simulink model "Tropfensimulation_x_y_Direction"  (R2025b)
settings: Solver=ode45  StartTime=0.0  StopTime=inf  RelTol=1e-6
values from neighbouring files (symbols this model uses):
  h0 = [0;3]    [Tropfensimulation_x_y_Direction_init.m]
  v0 = [7.5;0]    [Tropfensimulation_x_y_Direction_init.m]
libraries: simulink x1
settings Model: Creator=elmue  LastModifiedBy=ssokolov
settings SolverCC: AlgebraicLoopSolver=TrustRegion
settings DataIOCC: SaveFormat=StructureWithTime  OutputSaveName=xyout
settings DebuggingCC: UnconnectedInputMsg=warning  UnconnectedOutputMsg=warning  UnconnectedLineMsg=warning
settings ModelReferenceCC: EnableRefExpFcnMdlSchedulingChecks=on
settings RTWCC: GPUComputeCapability=3.5  DLArmComputeVersion=19.05

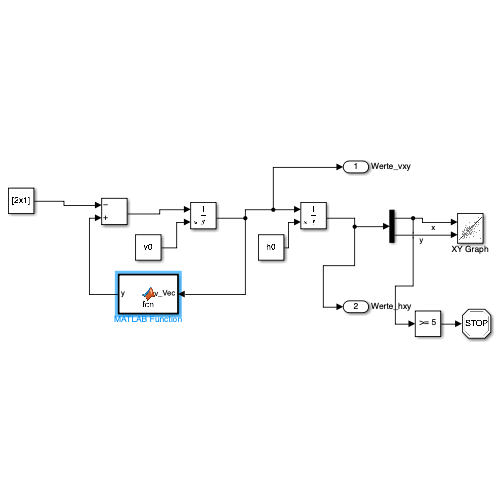
[thumbnail: Simulink's stored preview of the top-level diagram]
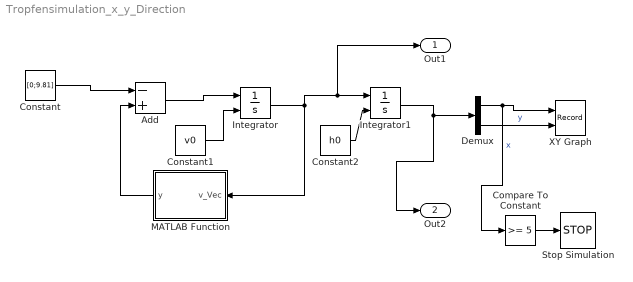
== system Tropfensimulation_x_y_Direction ==
  Add : Sum  Inputs=-+
  Compare To Constant : simulink/Logic and Bit Operations/Compare To Constant  relop=>=  const=5  OutDataTypeStr=boolean
  Constant : Constant  Value=[0;9.81]
  Constant1 : Constant  Value=v0
  Constant2 : Constant  Value=h0
  Demux : Demux  Outputs=2
  Integrator : Integrator  InitialConditionSource=external
  Integrator1 : Integrator  InitialConditionSource=external
  MATLAB Function : MATLAB Function  TreatAsAtomicUnit=on
  Stop Simulation : Stop
  XY Graph : Record  NumPorts=2.0  FileSettingsInternal="{\"entries\":[{\"content\":{\"excelSettings\":{\"content\":{},\"type\":\"Streamout.ExcelSettings\"},\"parquetSettings\":{\"content\":{},\"type\":\"Streamout.ParquetSettings\"}},\"type\":\"Streamout.FileSettingStorage\",\"uuid\":\"\"}],\"packageUris\":[\"http:\\/\\/schema.mathworks.com\\/mf0\\/streamout_blocks\\/R2020a\"],\"version\":\"1.0\"}"  FrameSettings=[0, 0]  Layout=[1 1]  SignalsInternal="{\"entries\":[{\"content\":{\"signals\":[{\"content\":{\"blockPath\":[],\"dimensions\":[1],\"domain\":\"\",\"lineColor\":\"#a2142f\",\"plots\":[ 1 ],\"port\":1,\"sid\":[\"\"],\"signalID\":1,\"signalName\":\"x\"},\"type\":\"RecordBlkView.Signal\",\"uuid\":\"\"},{\"content\":{\"blockPath\":[],\"dimensions\":[1],\"domain\":\"\",\"lineColor\":\"#139fff\",\"plots\":[ 1 ],\"port\":2,\"sid\":[\"\"],\"signalID\":2,\"signalName\":\"y\"},\"type\":\"RecordBlkView.Signal\",\"uuid\":\"\"}]},\"type\":\"RecordBlkView.InputSignals\",\"uuid\":\"\"}],\"packageUris\":[\"http:\\/\\/schema.mathworks.com\\/mf0\\/streamout_blocks\\/R2020a\"],\"version\":\"1.0\"}"  VisualizationBindings="{\"xyplotplugin\":{\"info\":[{\"series\":[{\"bindingParametersList\":[{\"parameter\":\"X-Axis\",\"signalID\":1,\"signalName\":\"x\"},{\"parameter\":\"Y-Axis\",\"signalID\":2,\"signalName\":\"y\"}],\"seriesID\":0}],\"subplotID\":1}]}}"  CompatibilityTag=XY  st=-1
  Out1 : Outport  SignalName=Werte_vxy
  Out2 : Outport  Port=2  SignalName=Werte_hxy
  wires:
  Integrator/1 -> Out1/1, Integrator1/1, MATLAB Function/1(v_Vec)
  Add/1 -> Integrator/1
  Constant/1 -> Add/1
  MATLAB Function/1(y) -> Add/2
  Constant1/1 -> Integrator/2
  Constant2/1 -> Integrator1/2
  Integrator1/1 -> Out2/1, Demux/1
  Demux/1 -> Compare To Constant/1, XY Graph/1  "x"
  Demux/2 -> XY Graph/2  "y"
  Compare To Constant/1 -> Stop Simulation/1

== matlab function Tropfensimulation_x_y_Direction/MATLAB Function ==
  data: v_Vec input; y output
function y = fcn(v_Vec)
vair=[15;0];
d=250*10^-6;
rhoair=1.225;
rhowater=1000;
vrel=vair-v_Vec;
cw=0.45;

m=d^3*rhowater*pi/6;
A=pi*d^2/4;

y=1./(2*m)*rhoair*A*cw.*vrel.*abs(vrel);
